simulink model "SeatBeltWarningSystem"  (R2022a)
settings: Solver=VariableStepAuto  StartTime=0.0  StopTime=inf  RelTol=1e-3
libraries: simulink x2
settings Model: Creator=dssan  LastModifiedBy=Sanjana_Bagewadi
settings SolverCC: AlgebraicLoopSolver=TrustRegion
settings DebuggingCC: UnconnectedInputMsg=warning  UnconnectedOutputMsg=warning  UnconnectedLineMsg=warning  SFMachineParentedDataDiag=warning
settings RTWCC: DLArmComputeVersion=19.05

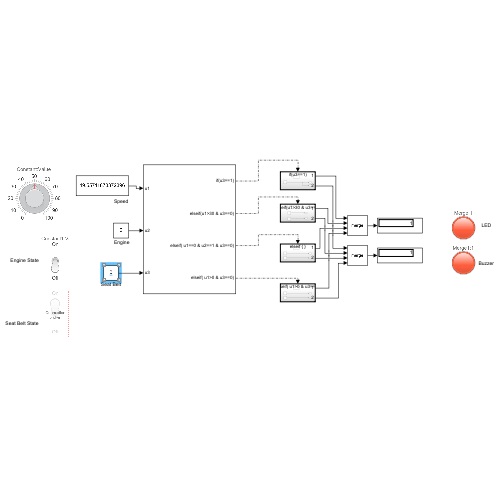
[thumbnail: Simulink's stored preview of the top-level diagram]
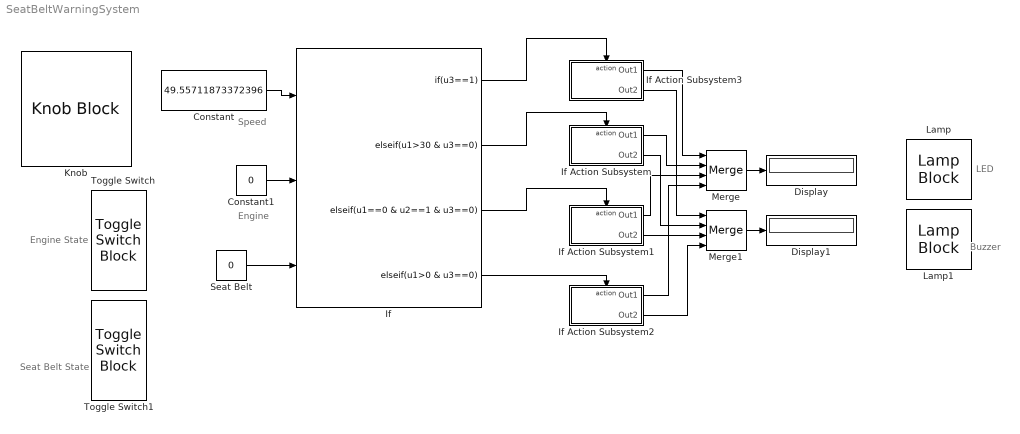
== system SeatBeltWarningSystem ==
  note: Seat Belt State
  note: Engine State
  note: Buzzer
  note: LED
  note: Engine
  note: Speed
  Constant : Constant  Value=49.55711873372396
  Constant1 : Constant  Value=0
  Display : Display
  Display1 : Display
  If : If  NumInputs=3  IfExpression=u3==1  ElseIfExpressions=u1>30 & u3==0, u1==0 & u2==1 & u3==0, u1>0 & u3==0  ShowElse=off
  If Action Subsystem : Subsystem  TreatAsAtomicUnit=on
  If Action Subsystem1 : Subsystem  TreatAsAtomicUnit=on
  If Action Subsystem2 : Subsystem  TreatAsAtomicUnit=on
  If Action Subsystem3 : Subsystem  TreatAsAtomicUnit=on
  Knob : KnobBlock
  Lamp : LampBlock
  Lamp1 : LampBlock
  Merge : Merge  Inputs=4
  Merge1 : Merge  Inputs=4
  Seat Belt : Constant  Value=0
  Toggle Switch : ToggleSwitchBlock
      settings: Values={{'Off', 'On'}, [0 1]}
  Toggle Switch1 : ToggleSwitchBlock
      settings: Values={{'Off', 'On'}, [0 1]}
  wires:
  Constant1/1 -> If/2
  Constant/1 -> If/1
  Merge1/1 -> Display1/1
  Merge/1 -> Display/1
  If Action Subsystem/1(Out1) -> Merge/2
  If Action Subsystem1/1(Out1) -> Merge/3
  If Action Subsystem/2(Out2) -> Merge1/2
  If Action Subsystem1/2(Out2) -> Merge1/3
  If/4 -> If Action Subsystem2/Action
  If/2 -> If Action Subsystem/Action
  If/1 -> If Action Subsystem3/Action
  If/3 -> If Action Subsystem1/Action
  If Action Subsystem3/1(Out1) -> Merge/1
  If Action Subsystem3/2(Out2) -> Merge1/1
  If Action Subsystem2/1(Out1) -> Merge/4
  If Action Subsystem2/2(Out2) -> Merge1/4
  Seat Belt/1 -> If/3

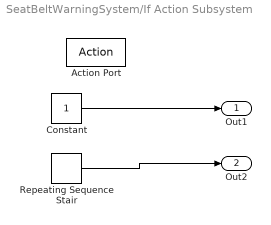
== system SeatBeltWarningSystem/If Action Subsystem ==
  Action Port : ActionPort  ActionPortLabel=elseif(u1>30 & u3==0)
  Constant : Constant
  Repeating Sequence Stair : simulink/Sources/Repeating Sequence Stair  OutValues=[0 1].'  tsamp=-1  OutMin=[]  OutMax=[]  OutDataTypeStr=double  OutputDataTypeScalingMode=double  OutDataType=fixdt(0,8)  ConRadixGroup=Best Precision: Vector-wise  OutScaling=2^-12
  Out1 : Outport
  Out2 : Outport  Port=2
  wires:
  Constant/1 -> Out1/1
  Repeating Sequence Stair/1 -> Out2/1

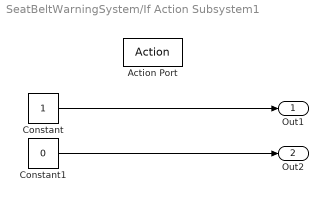
== system SeatBeltWarningSystem/If Action Subsystem1 ==
  Action Port : ActionPort  ActionPortLabel=elseif( u1==0 & u2==1 & u3==0)
  Constant : Constant
  Constant1 : Constant  Value=0
  Out1 : Outport
  Out2 : Outport  Port=2
  wires:
  Constant/1 -> Out1/1
  Constant1/1 -> Out2/1

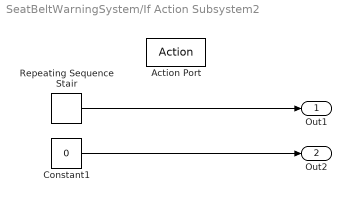
== system SeatBeltWarningSystem/If Action Subsystem2 ==
  Action Port : ActionPort  ActionPortLabel=elseif( u1>0 & u3==0)
  Constant1 : Constant  Value=0
  Repeating Sequence Stair : simulink/Sources/Repeating Sequence Stair  OutValues=[0 1].'  tsamp=-1  OutMin=[]  OutMax=[]  OutDataTypeStr=double  OutputDataTypeScalingMode=double  OutDataType=fixdt(0,8)  ConRadixGroup=Best Precision: Vector-wise  OutScaling=2^-12
  Out1 : Outport
  Out2 : Outport  Port=2
  wires:
  Repeating Sequence Stair/1 -> Out1/1
  Constant1/1 -> Out2/1

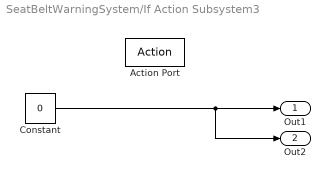
== system SeatBeltWarningSystem/If Action Subsystem3 ==
  Action Port : ActionPort  ActionPortLabel=if(u3==1)
  Constant : Constant  Value=0
  Out1 : Outport
  Out2 : Outport  Port=2
  wires:
  Constant/1 -> Out2/1, Out1/1
